simulink model "M182_Lab7ext"  (R2019b)
settings: Solver=VariableStepAuto  StartTime=0.0  StopTime=10.0  RelTol=1e-3
settings Model: Creator=scjcb  LastModifiedBy=scjcb

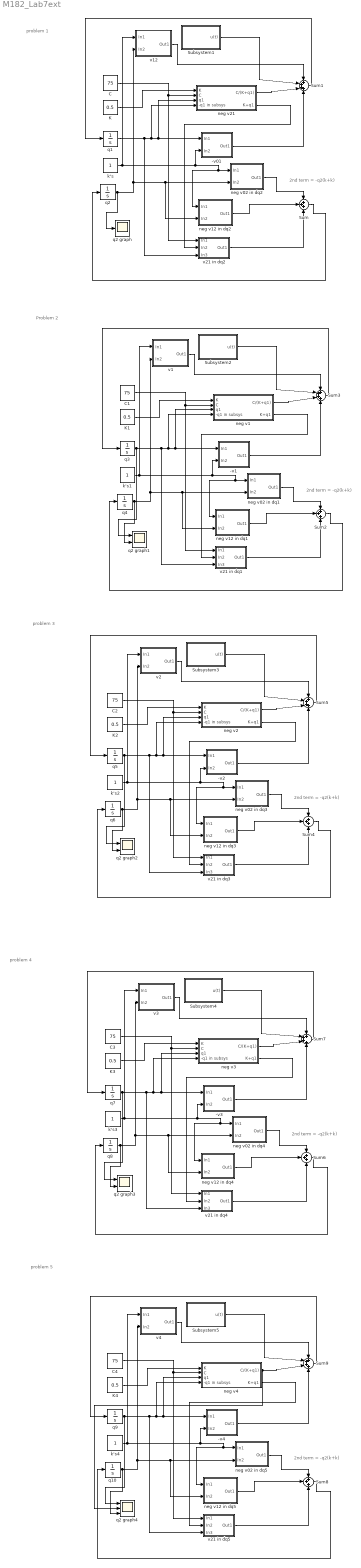
== system M182_Lab7ext ==
  note: problem 5
  note: problem 4
  note: problem 3
  note: problem 1
  note: Problem 2
  note: 2nd term = -q2(k+k)
  note: 2nd term = -q2(k+k)
  note: 2nd term = -q2(k+k)
  note: 2nd term = -q2(k+k)
  note: 2nd term = -q2(k+k)
  -v01 : Subsystem
  -v1 : Subsystem
  -v2 : Subsystem
  -v3 : Subsystem
  -v4 : Subsystem
  C{,1..4} (5 alike) : Constant  Value=75
  K{,1..4} (5 alike) : Constant  Value=0.5
  Subsystem1 : Subsystem
  Subsystem2 : Subsystem
  Subsystem3 : Subsystem
  Subsystem4 : Subsystem
  Subsystem5 : Subsystem
  Sum{,2,4,6,8} (5 alike) : Sum  Inputs=+++
  Sum{1,3,5,7,9} (5 alike) : Sum  Inputs=4
  k's{,1..4} (5 alike) : Constant
  neg v02 in dq1 : Subsystem
  neg v02 in dq2 : Subsystem
  neg v02 in dq3 : Subsystem
  neg v02 in dq4 : Subsystem
  neg v02 in dq5 : Subsystem
  neg v1 : Subsystem
  neg v12 in dq1 : Subsystem
  neg v12 in dq2 : Subsystem
  neg v12 in dq3 : Subsystem
  neg v12 in dq4 : Subsystem
  neg v12 in dq5 : Subsystem
  neg v2 : Subsystem
  neg v21 : Subsystem
  neg v3 : Subsystem
  neg v4 : Subsystem
  q{1..10} (10 alike) : Integrator
  q2 graph : Scope
  q2 graph1 : Scope  NumInputPorts=2
  q2 graph2 : Scope  NumInputPorts=2
  q2 graph3 : Scope  NumInputPorts=2
  q2 graph4 : Scope  NumInputPorts=3
  v1 : Subsystem
  v12 : Subsystem
  v2 : Subsystem
  v21 in dq1 : Subsystem
  v21 in dq2 : Subsystem
  v21 in dq3 : Subsystem
  v21 in dq4 : Subsystem
  v21 in dq5 : Subsystem
  v3 : Subsystem
  v4 : Subsystem
  wires:
  q1/1 -> v21 in dq2/3(In3), -v01/1(In1), neg v21/3(q1), neg v21/4(-q1 in subsys)
  C/1 -> v21 in dq2/1(In1), neg v21/2(C)
  k's/1 -> v12/1(In1), neg v12 in dq2/1(In1), neg v02 in dq2/1(In1), -v01/2(In2)
  q2/1 -> q2 graph/1, v12/2(In2), neg v12 in dq2/2(In2), neg v02 in dq2/2(In2)
  Sum1/1 -> q1/1
  Sum/1 -> q2/1
  K/1 -> neg v21/1(K)
  Subsystem1/1(u(t)) -> Sum1/2
  v12/1(Out1) -> Sum1/1
  neg v21/1(C/(K+q1)) -> Sum1/3
  -v01/1(Out1) -> Sum1/4
  neg v21/2(K+q1) -> v21 in dq2/2(In2)
  v21 in dq2/1(Out1) -> Sum/3
  neg v02 in dq2/1(Out1) -> Sum/1
  neg v12 in dq2/1(Out1) -> Sum/2
  neg v02 in dq1/1(Out1) -> Sum2/1
  K1/1 -> neg v1/1(K)
  Sum3/1 -> q3/1
  neg v12 in dq1/1(Out1) -> Sum2/2
  q4/1 -> q2 graph1/2, v1/2(In2), neg v12 in dq1/2(In2), neg v02 in dq1/2(In2)
  neg v1/2(K+q1) -> v21 in dq1/2(In2)
  v21 in dq1/1(Out1) -> Sum2/3
  -v1/1(Out1) -> Sum3/4
  v1/1(Out1) -> Sum3/1
  k's1/1 -> v1/1(In1), neg v12 in dq1/1(In1), neg v02 in dq1/1(In1), -v1/2(In2)
  neg v1/1(C/(K+q1)) -> Sum3/3
  q3/1 -> q2 graph1/1, v21 in dq1/3(In3), -v1/1(In1), neg v1/3(q1), neg v1/4(-q1 in subsys)
  Sum2/1 -> q4/1
  Subsystem2/1(u(t)) -> Sum3/2
  C1/1 -> v21 in dq1/1(In1), neg v1/2(C)
  C2/1 -> v21 in dq3/1(In1), neg v2/2(C)
  Subsystem3/1(u(t)) -> Sum5/2
  Sum4/1 -> q6/1
  q5/1 -> q2 graph2/1, v21 in dq3/3(In3), -v2/1(In1), neg v2/3(q1), neg v2/4(-q1 in subsys)
  v2/1(Out1) -> Sum5/1
  v21 in dq3/1(Out1) -> Sum4/3
  neg v2/1(C/(K+q1)) -> Sum5/3
  k's2/1 -> v2/1(In1), neg v12 in dq3/1(In1), neg v02 in dq3/1(In1), -v2/2(In2)
  q6/1 -> q2 graph2/2, v2/2(In2), neg v12 in dq3/2(In2), neg v02 in dq3/2(In2)
  neg v02 in dq3/1(Out1) -> Sum4/1
  -v2/1(Out1) -> Sum5/4
  Sum5/1 -> q5/1
  neg v2/2(K+q1) -> v21 in dq3/2(In2)
  neg v12 in dq3/1(Out1) -> Sum4/2
  K2/1 -> neg v2/1(K)
  neg v3/1(C/(K+q1)) -> Sum7/3
  v21 in dq4/1(Out1) -> Sum6/3
  v3/1(Out1) -> Sum7/1
  q7/1 -> q2 graph3/1, v21 in dq4/3(In3), -v3/1(In1), neg v3/3(q1), neg v3/4(-q1 in subsys)
  Sum6/1 -> q8/1
  Subsystem4/1(u(t)) -> Sum7/2
  neg v3/2(K+q1) -> v21 in dq4/2(In2)
  Sum7/1 -> q7/1
  neg v02 in dq4/1(Out1) -> Sum6/1
  -v3/1(Out1) -> Sum7/4
  q8/1 -> q2 graph3/2, v3/2(In2), neg v12 in dq4/2(In2), neg v02 in dq4/2(In2)
  neg v12 in dq4/1(Out1) -> Sum6/2
  C3/1 -> v21 in dq4/1(In1), neg v3/2(C)
  k's3/1 -> v3/1(In1), neg v12 in dq4/1(In1), neg v02 in dq4/1(In1), -v3/2(In2)
  K3/1 -> neg v3/1(K)
  K4/1 -> neg v4/1(K)
  k's4/1 -> v4/1(In1), neg v12 in dq5/1(In1), neg v02 in dq5/1(In1), -v4/2(In2)
  neg v12 in dq5/1(Out1) -> Sum8/2
  C4/1 -> v21 in dq5/1(In1), neg v4/2(C)
  q10/1 -> q2 graph4/3, v4/2(In2), neg v12 in dq5/2(In2), neg v02 in dq5/2(In2)
  neg v4/2(K+q1) -> v21 in dq5/2(In2)
  Subsystem5/1(u(t)) -> Sum9/2
  -v4/1(Out1) -> Sum9/4
  Sum8/1 -> q10/1
  Sum9/1 -> q9/1
  q9/1 -> q2 graph4/1, v21 in dq5/3(In3), -v4/1(In1), neg v4/3(q1), neg v4/4(-q1 in subsys)
  neg v02 in dq5/1(Out1) -> Sum8/1
  v4/1(Out1) -> Sum9/1
  neg v4/1(C/(K+q1)) -> q2 graph4/2, Sum9/3
  v21 in dq5/1(Out1) -> Sum8/3

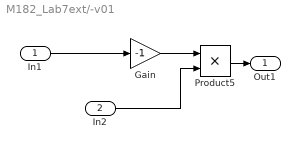
== system M182_Lab7ext/-v01 ==
  In1 : Inport
  In2 : Inport  Port=2
  Gain : Gain  Gain=-1
  Product5 : Product  Inputs=**
  Out1 : Outport
  wires:
  In1/1 -> Gain/1
  Product5/1 -> Out1/1
  Gain/1 -> Product5/1
  In2/1 -> Product5/2

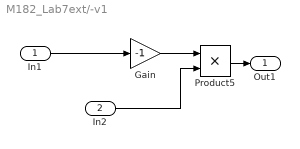
== system M182_Lab7ext/-v1 ==
  In1 : Inport
  In2 : Inport  Port=2
  Gain : Gain  Gain=-1
  Product5 : Product  Inputs=**
  Out1 : Outport
  wires:
  In1/1 -> Gain/1
  Product5/1 -> Out1/1
  Gain/1 -> Product5/1
  In2/1 -> Product5/2

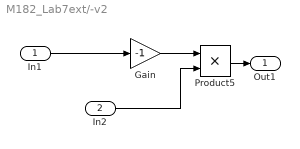
== system M182_Lab7ext/-v2 ==
  In1 : Inport
  In2 : Inport  Port=2
  Gain : Gain  Gain=-1
  Product5 : Product  Inputs=**
  Out1 : Outport
  wires:
  In1/1 -> Gain/1
  Product5/1 -> Out1/1
  Gain/1 -> Product5/1
  In2/1 -> Product5/2

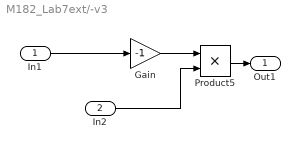
== system M182_Lab7ext/-v3 ==
  In1 : Inport
  In2 : Inport  Port=2
  Gain : Gain  Gain=-1
  Product5 : Product  Inputs=**
  Out1 : Outport
  wires:
  In1/1 -> Gain/1
  Product5/1 -> Out1/1
  Gain/1 -> Product5/1
  In2/1 -> Product5/2

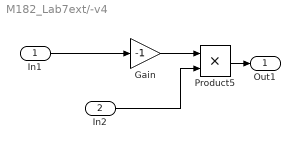
== system M182_Lab7ext/-v4 ==
  In1 : Inport
  In2 : Inport  Port=2
  Gain : Gain  Gain=-1
  Product5 : Product  Inputs=**
  Out1 : Outport
  wires:
  In1/1 -> Gain/1
  Product5/1 -> Out1/1
  Gain/1 -> Product5/1
  In2/1 -> Product5/2

== system M182_Lab7ext/Subsystem1 ==
  note: D as gain
  note: 1(t) = Step
  Gain2 : Gain
  Step : Step  Time=0  SampleTime=0
  u(t) : Outport
  wires:
  Step/1 -> Gain2/1
  Gain2/1 -> u(t)/1

== system M182_Lab7ext/Subsystem2 ==
  note: D as gain
  note: 1(t) = Step
  Gain2 : Gain  Gain=[1,2,4]
  Step : Step  Time=0  SampleTime=0
  u(t) : Outport
  wires:
  Step/1 -> Gain2/1
  Gain2/1 -> u(t)/1

== system M182_Lab7ext/Subsystem3 ==
  note: D as gain
  note: 1(t) = Step
  Gain2 : Gain  Gain=[40,80,160]
  Step : Step  Time=0  SampleTime=0
  u(t) : Outport
  wires:
  Step/1 -> Gain2/1
  Gain2/1 -> u(t)/1

== system M182_Lab7ext/Subsystem4 ==
  note: D as gain
  note: 1(t) = Step
  Gain2 : Gain  Gain=[100,200,400]
  Step : Step  Time=0  SampleTime=0
  u(t) : Outport
  wires:
  Step/1 -> Gain2/1
  Gain2/1 -> u(t)/1

== system M182_Lab7ext/Subsystem5 ==
  note: D as gain
  note: 1(t) = Step
  Gain2 : Gain  Gain=[40,80,160]
  Step : Step  Time=0  SampleTime=0
  u(t) : Outport
  wires:
  Step/1 -> Gain2/1
  Gain2/1 -> u(t)/1

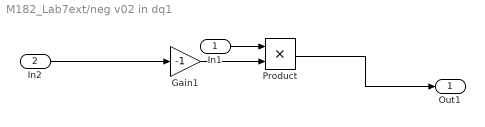
== system M182_Lab7ext/neg v02 in dq1 ==
  In1 : Inport
  In2 : Inport  Port=2
  Gain1 : Gain  Gain=-1
  Product : Product
  Out1 : Outport
  wires:
  Gain1/1 -> Product/2
  In2/1 -> Gain1/1
  Product/1 -> Out1/1
  In1/1 -> Product/1

== system M182_Lab7ext/neg v02 in dq2 ==
  In1 : Inport
  In2 : Inport  Port=2
  Gain1 : Gain  Gain=-1
  Product : Product
  Out1 : Outport
  wires:
  Gain1/1 -> Product/2
  In2/1 -> Gain1/1
  Product/1 -> Out1/1
  In1/1 -> Product/1

== system M182_Lab7ext/neg v02 in dq3 ==
  In1 : Inport
  In2 : Inport  Port=2
  Gain1 : Gain  Gain=-1
  Product : Product
  Out1 : Outport
  wires:
  Gain1/1 -> Product/2
  In2/1 -> Gain1/1
  Product/1 -> Out1/1
  In1/1 -> Product/1

== system M182_Lab7ext/neg v02 in dq4 ==
  In1 : Inport
  In2 : Inport  Port=2
  Gain1 : Gain  Gain=-1
  Product : Product
  Out1 : Outport
  wires:
  Gain1/1 -> Product/2
  In2/1 -> Gain1/1
  Product/1 -> Out1/1
  In1/1 -> Product/1

== system M182_Lab7ext/neg v02 in dq5 ==
  In1 : Inport
  In2 : Inport  Port=2
  Gain1 : Gain  Gain=-1
  Product : Product
  Out1 : Outport
  wires:
  Gain1/1 -> Product/2
  In2/1 -> Gain1/1
  Product/1 -> Out1/1
  In1/1 -> Product/1

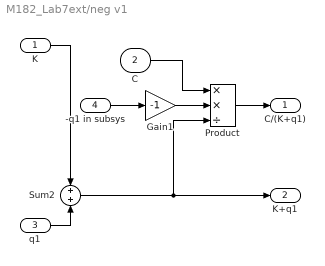
== system M182_Lab7ext/neg v1 ==
  K : Inport
  C : Inport  Port=2
  q1 : Inport  Port=3
  -q1 in subsys : Inport  Port=4
  Gain1 : Gain  Gain=-1
  Product : Product  Inputs=**/
  Sum2 : Sum
  C/(K+q1) : Outport
  K+q1 : Outport  Port=2
  wires:
  Sum2/1 -> Product/3, K+q1/1
  q1/1 -> Sum2/2
  K/1 -> Sum2/1
  Product/1 -> C/(K+q1)/1
  C/1 -> Product/1
  -q1 in subsys/1 -> Gain1/1
  Gain1/1 -> Product/2

== system M182_Lab7ext/neg v12 in dq1 ==
  In1 : Inport
  In2 : Inport  Port=2
  Gain : Gain  Gain=-1
  Product1 : Product
  Out1 : Outport
  wires:
  Gain/1 -> Product1/1
  Product1/1 -> Out1/1
  In1/1 -> Product1/2
  In2/1 -> Gain/1

== system M182_Lab7ext/neg v12 in dq2 ==
  In1 : Inport
  In2 : Inport  Port=2
  Gain : Gain  Gain=-1
  Product1 : Product
  Out1 : Outport
  wires:
  Gain/1 -> Product1/1
  Product1/1 -> Out1/1
  In1/1 -> Product1/2
  In2/1 -> Gain/1

== system M182_Lab7ext/neg v12 in dq3 ==
  In1 : Inport
  In2 : Inport  Port=2
  Gain : Gain  Gain=-1
  Product1 : Product
  Out1 : Outport
  wires:
  Gain/1 -> Product1/1
  Product1/1 -> Out1/1
  In1/1 -> Product1/2
  In2/1 -> Gain/1

== system M182_Lab7ext/neg v12 in dq4 ==
  In1 : Inport
  In2 : Inport  Port=2
  Gain : Gain  Gain=-1
  Product1 : Product
  Out1 : Outport
  wires:
  Gain/1 -> Product1/1
  Product1/1 -> Out1/1
  In1/1 -> Product1/2
  In2/1 -> Gain/1

== system M182_Lab7ext/neg v12 in dq5 ==
  In1 : Inport
  In2 : Inport  Port=2
  Gain : Gain  Gain=-1
  Product1 : Product
  Out1 : Outport
  wires:
  Gain/1 -> Product1/1
  Product1/1 -> Out1/1
  In1/1 -> Product1/2
  In2/1 -> Gain/1

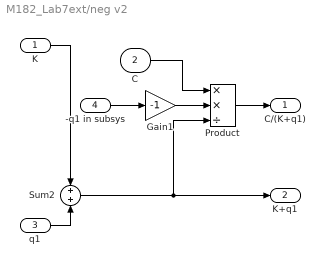
== system M182_Lab7ext/neg v2 ==
  K : Inport
  C : Inport  Port=2
  q1 : Inport  Port=3
  -q1 in subsys : Inport  Port=4
  Gain1 : Gain  Gain=-1
  Product : Product  Inputs=**/
  Sum2 : Sum
  C/(K+q1) : Outport
  K+q1 : Outport  Port=2
  wires:
  Sum2/1 -> Product/3, K+q1/1
  q1/1 -> Sum2/2
  K/1 -> Sum2/1
  Product/1 -> C/(K+q1)/1
  C/1 -> Product/1
  -q1 in subsys/1 -> Gain1/1
  Gain1/1 -> Product/2

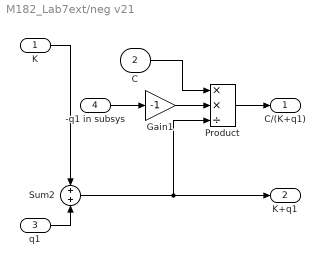
== system M182_Lab7ext/neg v21 ==
  K : Inport
  C : Inport  Port=2
  q1 : Inport  Port=3
  -q1 in subsys : Inport  Port=4
  Gain1 : Gain  Gain=-1
  Product : Product  Inputs=**/
  Sum2 : Sum
  C/(K+q1) : Outport
  K+q1 : Outport  Port=2
  wires:
  Sum2/1 -> Product/3, K+q1/1
  q1/1 -> Sum2/2
  K/1 -> Sum2/1
  Product/1 -> C/(K+q1)/1
  C/1 -> Product/1
  -q1 in subsys/1 -> Gain1/1
  Gain1/1 -> Product/2

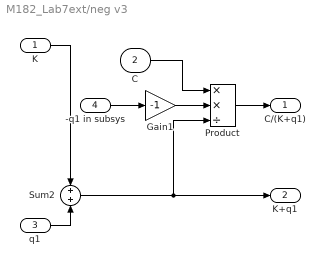
== system M182_Lab7ext/neg v3 ==
  K : Inport
  C : Inport  Port=2
  q1 : Inport  Port=3
  -q1 in subsys : Inport  Port=4
  Gain1 : Gain  Gain=-1
  Product : Product  Inputs=**/
  Sum2 : Sum
  C/(K+q1) : Outport
  K+q1 : Outport  Port=2
  wires:
  Sum2/1 -> Product/3, K+q1/1
  q1/1 -> Sum2/2
  K/1 -> Sum2/1
  Product/1 -> C/(K+q1)/1
  C/1 -> Product/1
  -q1 in subsys/1 -> Gain1/1
  Gain1/1 -> Product/2

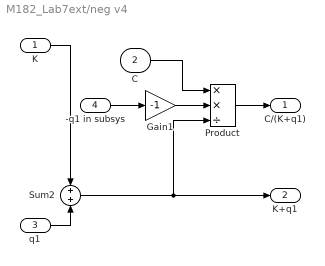
== system M182_Lab7ext/neg v4 ==
  K : Inport
  C : Inport  Port=2
  q1 : Inport  Port=3
  -q1 in subsys : Inport  Port=4
  Gain1 : Gain  Gain=-1
  Product : Product  Inputs=**/
  Sum2 : Sum
  C/(K+q1) : Outport
  K+q1 : Outport  Port=2
  wires:
  Sum2/1 -> Product/3, K+q1/1
  q1/1 -> Sum2/2
  K/1 -> Sum2/1
  Product/1 -> C/(K+q1)/1
  C/1 -> Product/1
  -q1 in subsys/1 -> Gain1/1
  Gain1/1 -> Product/2

== system M182_Lab7ext/v1 ==
  In1 : Inport
  In2 : Inport  Port=2
  Product2 : Product  Inputs=**
  Out1 : Outport
  wires:
  In2/1 -> Product2/2
  In1/1 -> Product2/1
  Product2/1 -> Out1/1

== system M182_Lab7ext/v12 ==
  In1 : Inport
  In2 : Inport  Port=2
  Product2 : Product  Inputs=**
  Out1 : Outport
  wires:
  In2/1 -> Product2/2
  In1/1 -> Product2/1
  Product2/1 -> Out1/1

== system M182_Lab7ext/v2 ==
  In1 : Inport
  In2 : Inport  Port=2
  Product2 : Product  Inputs=**
  Out1 : Outport
  wires:
  In2/1 -> Product2/2
  In1/1 -> Product2/1
  Product2/1 -> Out1/1

== system M182_Lab7ext/v21 in dq1 ==
  In1 : Inport
  In2 : Inport  Port=2
  In3 : Inport  Port=3
  Product3 : Product  Inputs=**/
  Out1 : Outport
  wires:
  Product3/1 -> Out1/1
  In1/1 -> Product3/2
  In3/1 -> Product3/1
  In2/1 -> Product3/3

== system M182_Lab7ext/v21 in dq2 ==
  In1 : Inport
  In2 : Inport  Port=2
  In3 : Inport  Port=3
  Product3 : Product  Inputs=**/
  Out1 : Outport
  wires:
  Product3/1 -> Out1/1
  In1/1 -> Product3/2
  In3/1 -> Product3/1
  In2/1 -> Product3/3

== system M182_Lab7ext/v21 in dq3 ==
  In1 : Inport
  In2 : Inport  Port=2
  In3 : Inport  Port=3
  Product3 : Product  Inputs=**/
  Out1 : Outport
  wires:
  Product3/1 -> Out1/1
  In1/1 -> Product3/2
  In3/1 -> Product3/1
  In2/1 -> Product3/3

== system M182_Lab7ext/v21 in dq4 ==
  In1 : Inport
  In2 : Inport  Port=2
  In3 : Inport  Port=3
  Product3 : Product  Inputs=**/
  Out1 : Outport
  wires:
  Product3/1 -> Out1/1
  In1/1 -> Product3/2
  In3/1 -> Product3/1
  In2/1 -> Product3/3

== system M182_Lab7ext/v21 in dq5 ==
  In1 : Inport
  In2 : Inport  Port=2
  In3 : Inport  Port=3
  Product3 : Product  Inputs=**/
  Out1 : Outport
  wires:
  Product3/1 -> Out1/1
  In1/1 -> Product3/2
  In3/1 -> Product3/1
  In2/1 -> Product3/3

== system M182_Lab7ext/v3 ==
  In1 : Inport
  In2 : Inport  Port=2
  Product2 : Product  Inputs=**
  Out1 : Outport
  wires:
  In2/1 -> Product2/2
  In1/1 -> Product2/1
  Product2/1 -> Out1/1

== system M182_Lab7ext/v4 ==
  In1 : Inport
  In2 : Inport  Port=2
  Product2 : Product  Inputs=**
  Out1 : Outport
  wires:
  In2/1 -> Product2/2
  In1/1 -> Product2/1
  Product2/1 -> Out1/1
